simulink model "comWiperCtrlUnit"  (R2023b)
settings: Solver=FixedStepAuto  StartTime=0.0  StopTime=10.0  RelTol=1e-3  EnableMultiTasking=on
model workspace (MAT data in the model file):
  bladeLength = Simulink.Parameter
  bladeLength.Value = 0.5
  bladeLength.Complexity = 'real'
  bladeLength.Dimensions = [1 1]
  bladeLength.DataType = 'double'
  bladeMass = Simulink.Parameter
  bladeMass.Value = 0.3
  bladeMass.Complexity = 'real'
  bladeMass.Dimensions = [1 1]
  bladeMass.DataType = 'double'
  inertMoment = Simulink.Parameter
  inertMoment.Value = 0.6
  inertMoment.Complexity = 'real'
  inertMoment.Dimensions = [1 1]
  inertMoment.DataType = 'double'
  sweepAngle = Simulink.Parameter
  sweepAngle.Value = 120
  sweepAngle.Complexity = 'real'
  sweepAngle.Dimensions = [1 1]
  sweepAngle.DataType = 'double'
undefined symbols (not defined in the file or in its folder): motor, position
settings Model: DataDictionary=prdLuxuryCar_dict.sldd  ParameterArgumentNames=bladeLength,bladeMass,inertMoment,sweepAngle  Creator=DucHM28  LastModifiedBy=DucHM28
settings OptimizationCC: DefaultParameterBehavior=Inlined  OptimizeBlockIOStorage=off  EnhancedBackFolding=on  PassReuseOutputArgsThreshold=0  ZeroExternalMemoryAtStartup=off  ZeroInternalMemoryAtStartup=off  OptimizeDataStoreBuffers=off  BusAssignmentInplaceUpdate=off
settings DebuggingCC: ParameterTunabilityLossMsg=error  SFUnexpectedBacktrackingDiag=warning  SFNoUnconditionalDefaultTransitionDiag=warning
settings SFSimCC: MATLABDynamicMemAlloc=off
settings RTWCC: GenerateReport=on  BuildConfiguration=Debug  LaunchReport=on  TargetLang=C++  GPUComputeCapability=5.0
settings CodeAppCC: ForceParamTrailComments=on  OperatorAnnotations=on  MATLABSourceComments=on  EnableCustomComments=on
settings GRTTargetCC: TargetLangStandard=C++11 (ISO)  CombineSignalStateStructs=on  CodeInterfacePackaging=C++ class  SupportVariableSizeSignals=on  MultiInstanceErrorCode=Warning

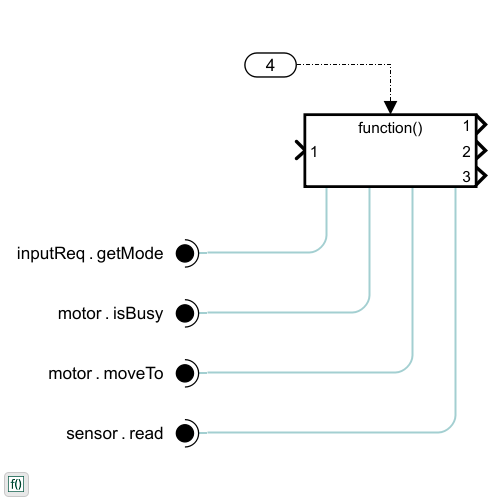
[thumbnail: Simulink's stored preview of the top-level diagram]
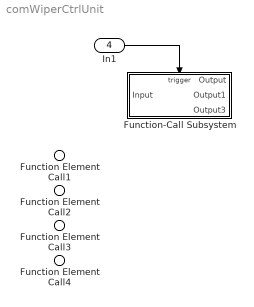
== system comWiperCtrlUnit ==
  Function Element Call1 : Inport  AllowServiceAccess=on  PortName=inputReq  Element=getMode
  Function Element Call3 : Inport  Port=2  AllowServiceAccess=on  PortName=motor  Element=moveTo
  Function Element Call2 : Inport  Port=2  AllowServiceAccess=on  PortName=motor  Element=isBusy
  Function Element Call4 : Inport  Port=3  AllowServiceAccess=on  PortName=sensor  Element=read
  In1 : Inport  Port=4  OutputFunctionCall=on
  Function-Call Subsystem : Subsystem  TreatAsAtomicUnit=on
  wires:
  In1/1 -> Function-Call Subsystem/Trigger

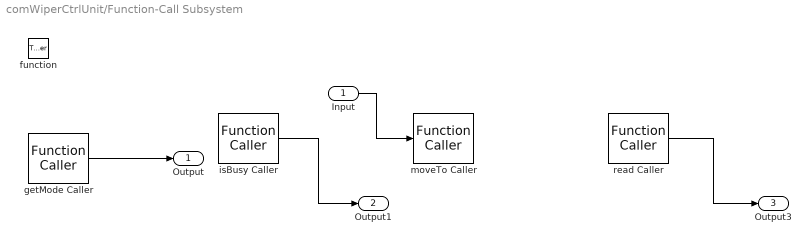
== system comWiperCtrlUnit/Function-Call Subsystem ==
  Input : Inport
  function : TriggerPort  TriggerType=function-call  VariantControl=(inherit)
  getMode Caller : FunctionCaller  FunctionPrototype=y = inputReq.getMode()  InputArgumentSpecifications=<Enter example>  OutputArgumentSpecifications=<Enter example>
  isBusy Caller : FunctionCaller  FunctionPrototype=y = motor.isBusy()  InputArgumentSpecifications=<Enter example>  OutputArgumentSpecifications=<Enter example>
  moveTo Caller : FunctionCaller  FunctionPrototype=motor.moveTo(position)  InputArgumentSpecifications=<Enter example>  OutputArgumentSpecifications=<Enter example>
  read Caller : FunctionCaller  FunctionPrototype=y = sensor.read()  InputArgumentSpecifications=<Enter example>  OutputArgumentSpecifications=<Enter example>
  Output : Outport
  Output1 : Outport  Port=2
  Output3 : Outport  Port=3
  wires:
  getMode Caller/1 -> Output/1
  isBusy Caller/1 -> Output1/1
  read Caller/1 -> Output3/1
  Input/1 -> moveTo Caller/1
